simulink library "TBMPC_Blocks"  (R2020a)
settings: Solver=VariableStepAuto  StartTime=0.0  StopTime=10.0  RelTol=1e-3
values from neighbouring files (symbols this model uses):
  L = [-K eye(2)]*M_theta    [following_paper_example.m]
  Q = 10*eye(6)    [TRMPC_initializer.m]    (also in following_paper_example.m = eye(2))
undefined symbols (not defined in the file or in its folder): A_timeshift, Ad, Aeq, Bd, beq, K_feedback, x_mes_guess
settings Model: Creator=hough  LastModifiedBy=hough

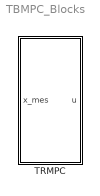
== system TBMPC_Blocks ==
  TRMPC : Subsystem

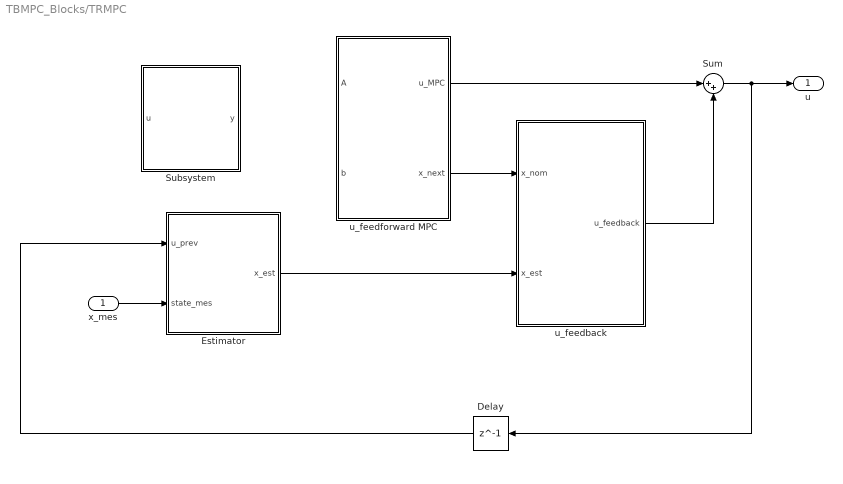
== system TBMPC_Blocks/TRMPC ==
  x_mes : Inport
  Delay : Delay  DelayLength=1
  Estimator : Subsystem
  Subsystem : Subsystem
  Sum : Sum  Inputs=|++
  u_feedback : Subsystem
  u_feedforward MPC : Subsystem
  u : Outport
  wires:
  Delay/1 -> Estimator/1(u_prev)
  u_feedforward MPC/1(u_MPC) -> Sum/1
  Sum/1 -> u/1, Delay/1
  Estimator/1(x_est) -> u_feedback/2(x_est)
  u_feedforward MPC/2(x_next) -> u_feedback/1(x_nom)
  x_mes/1 -> Estimator/2(state_mes)
  u_feedback/1(u_feedback) -> Sum/2

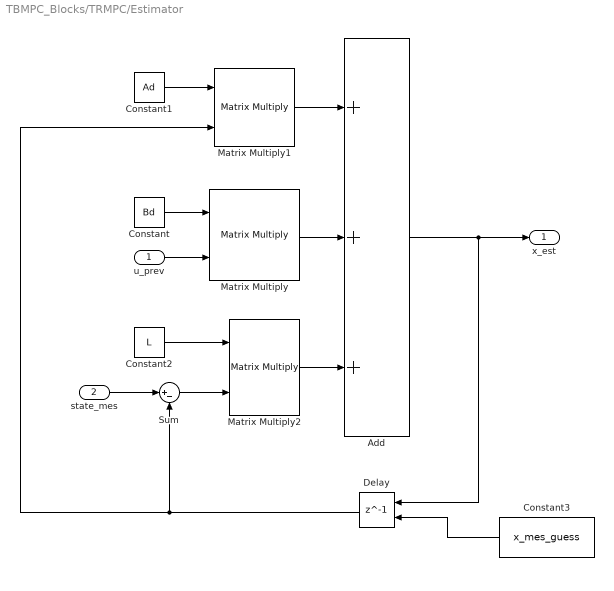
== system TBMPC_Blocks/TRMPC/Estimator ==
  u_prev : Inport
  state_mes : Inport  Port=2
  Add : Sum  Inputs=+++
  Constant : Constant  Value=Bd
  Constant1 : Constant  Value=Ad
  Constant2 : Constant  Value=L
  Constant3 : Constant  Value=x_mes_guess
  Delay : Delay  DelayLength=1  InitialConditionSource=Input port  InitialCondition=x_mes_guess
      settings: InputPortMap=u0,p4
  Matrix Multiply : Product  Multiplication=Matrix(*)
  Matrix Multiply1 : Product  Multiplication=Matrix(*)
  Matrix Multiply2 : Product  Multiplication=Matrix(*)
  Sum : Sum  Inputs=|+-
  x_est : Outport
  wires:
  u_prev/1 -> Matrix Multiply/2
  Constant/1 -> Matrix Multiply/1
  Constant1/1 -> Matrix Multiply1/1
  Constant2/1 -> Matrix Multiply2/1
  Sum/1 -> Matrix Multiply2/2
  state_mes/1 -> Sum/1
  Matrix Multiply/1 -> Add/2
  Matrix Multiply1/1 -> Add/1
  Matrix Multiply2/1 -> Add/3
  Add/1 -> Delay/1, x_est/1
  Delay/1 -> Sum/2, Matrix Multiply1/2
  Constant3/1 -> Delay/2

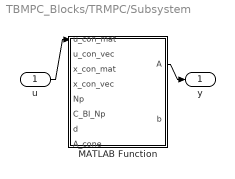
== system TBMPC_Blocks/TRMPC/Subsystem ==
  u : Inport
  MATLAB Function : MATLAB Function  TreatAsAtomicUnit=on
  y : Outport
  wires:
  MATLAB Function/1(A) -> y/1
  u/1 -> MATLAB Function/1(u_con_mat)

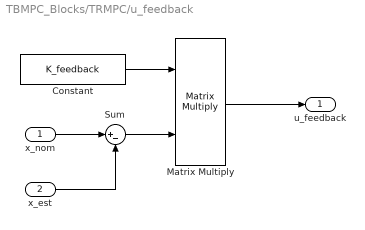
== system TBMPC_Blocks/TRMPC/u_feedback ==
  x_nom : Inport
  x_est : Inport  Port=2
  Constant : Constant  Value=K_feedback
  Matrix Multiply : Product  Multiplication=Matrix(*)
  Sum : Sum  Inputs=|+-
  u_feedback : Outport
  wires:
  x_nom/1 -> Sum/1
  x_est/1 -> Sum/2
  Sum/1 -> Matrix Multiply/2
  Constant/1 -> Matrix Multiply/1
  Matrix Multiply/1 -> u_feedback/1

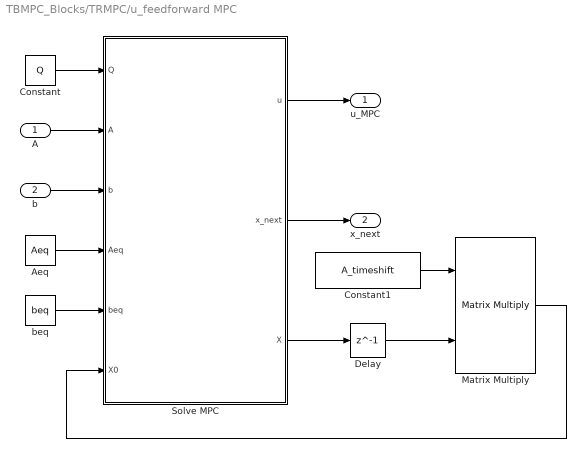
== system TBMPC_Blocks/TRMPC/u_feedforward MPC ==
  A : Inport
  b : Inport  Port=2
  Aeq : Constant  Value=Aeq
  Constant : Constant  Value=Q
  Constant1 : Constant  Value=A_timeshift
  Delay : Delay  DelayLength=1
  Matrix Multiply : Product  Multiplication=Matrix(*)
  Solve MPC : MATLAB Function  TreatAsAtomicUnit=on
  beq : Constant  Value=beq
  u_MPC : Outport
  x_next : Outport  Port=2
  wires:
  A/1 -> Solve MPC/2(A)
  Matrix Multiply/1 -> Solve MPC/6(X0)
  beq/1 -> Solve MPC/5(beq)
  Constant1/1 -> Matrix Multiply/1
  Constant/1 -> Solve MPC/1(Q)
  Delay/1 -> Matrix Multiply/2
  Aeq/1 -> Solve MPC/4(Aeq)
  b/1 -> Solve MPC/3(b)
  Solve MPC/3(X) -> Delay/1
  Solve MPC/1(u) -> u_MPC/1
  Solve MPC/2(x_next) -> x_next/1

== matlab function TBMPC_Blocks/TRMPC/Subsystem/MATLAB Function ==
  data: u_con_mat input; A output; u_con_vec input; x_con_mat input; x_con_vec input; Np input; C_BI_Np input; d input; A_cone input; b output
function [A, b] = fcn(u_con_mat, u_con_vec, x_con_mat, x_con_vec, Np, C_BI_Np, d, A_cone)

    [A, b] = return_inequality_con_mat_and_vec(u_con_mat, u_con_vec, x_con_mat, x_con_vec, Np, [], [], C_BI_Np, d, A_cone)

end

== matlab function TBMPC_Blocks/TRMPC/u_feedforward MPC/Solve MPC ==
  data: Q input; u output; x_next output; A input; b input; Aeq input; beq input; X0 input; X output
function [u, x_next, X] = MPC(Q, A, b, Aeq, beq, X0)

    % solve the full time-horizon (states + inputs)
    options = optimoptions('quadprog','Display','none');
    X = quadprog(Q, [], A, b, Aeq, beq, [], [], X0, options);

    % get the input only (first timestep)
    u = X(1:3);
    
    % get the next desired state (3 for vel, 3 for pos)
    x_next = X(4:10);
    
end
